simulink model "rtwdemo_sil"  (Simulink 6.0)
settings: Solver=ode3  StartTime=0.0  StopTime=5  FixedStep=.01  RelTol=1e-3
libraries: rtwdemowidgets x1
CloseFcn:
  | rtwprivate ssgencode ModelCloseRequest rtwdemo_sil
settings Model: Creator=The MathWorks Inc.  LastModifiedBy=batserve  ExtModeAutoUpdateStatusClock=off
settings DataIOCC: SaveOutput=off  SaveTime=off  SignalLoggingName=sigsOut
settings OptimizationCC: InlineParams=on  EnforceIntegerDowncast=off  StateBitsets=on  DataBitsets=on  UseTempVars=on  NoFixptDivByZeroProtection=on  LifeSpan=1
settings DebuggingCC: CheckExecutionContextPreStartOutputMsg=on  CheckExecutionContextRuntimeOutputMsg=on  SolverPrmCheckMsg=none
settings RTWCC: SystemTargetFile=ert.tlc  TemplateMakefile=ert_default_tmf  GenerateReport=on  RTWVerbose=off  ProcessScript=ert_make_rtw_hook  IncludeHyperlinkInReport=on  LaunchReport=on
settings CodeAppCC: ForceParamTrailComments=on  IgnoreCustomStorageClasses=off  SimulinkDataObjDesc=on  CustomSymbolStr=$N$M  InsertBlockDesc=on
settings ERTTargetCC: TargetFcnLib=ansi_tfl_tmw.mat  GenFloatMathFcnCalls=ANSI_C  GenerateSampleERTMain=on  IncludeMdlTerminateFcn=off  SupportComplex=off  SupportContinuousTime=on  GenerateErtSFunction=on  InlinedParameterPlacement=NonHierarchical  RootIOFormat=Individual Arguments  ERTCustomFileTemplate=example_file_process.tlc  InitialValueSource=Model

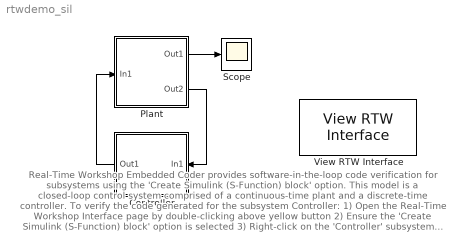
== system rtwdemo_sil ==
  note: Real-Time Workshop Embedded Coder provides software-in-the-loop code verification for subsystems
      | using the 'Create Simulink (S-Function) block' option.  This model is a closed-loop control
      | system comprised of a continuous-time plant and a discrete-time controller.
      |
      | To verify the code generated for the subsystem Controller:
      |
      | 1) Open the Real-Time Workshop Interface page by double-clicking above yellow button
      | 2) Ensure the 'Create Simulink (S-Function) block' option is selected
      | 3) Right-click on the 'Controller' subsystem and select Real-Time Workshop->Build Subsystem...
      | 4) Press the 'Build' button once the parameter dialog appears
      |
      | An S-Function block is created in an untitled library.  This S-Function is a wrapper for the
      | generated subsystem code, and can be used to verify the code provides the same result as the
      | original subsystem.  Replace the original system with the S-Function block and re-run the
      | simulation to verify the output is correct.
  Controller : Subsystem  Orientation=left  TreatAsAtomicUnit=on  PropExecContextAcrossSSBoundary=on
      settings: RTWFcnNameOpts=Use subsystem name  RTWFileNameOpts=Use function name
  Plant : Subsystem  PropExecContextAcrossSSBoundary=on
  Scope : Scope
      settings: TimeRange=5  YMin=0  YMax=10
  View RTW Interface : rtwdemowidgets/View RTW Interface
  wires:
  Controller/1(Out1) -> Plant/1(In1)
  Plant/1(Out1) -> Scope/1
  Plant/2(Out2) -> Controller/1(In1)

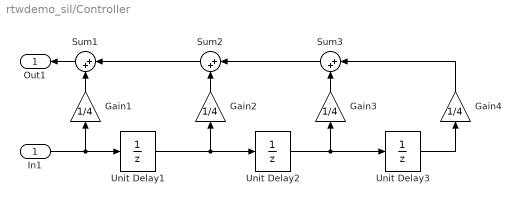
== system rtwdemo_sil/Controller ==
  In1 : Inport  Port=1  SampleTime=.01  LatchInput=off
  Gain{1..4} (4 alike) : Gain  Orientation=up  Gain=1/4  SaturateOnIntegerOverflow=on
  Sum1 : Sum  Orientation=left  Inputs=|++  SaturateOnIntegerOverflow=on  InputSameDT=on
  Sum2 : Sum  Orientation=left  Inputs=|++  SaturateOnIntegerOverflow=on  InputSameDT=on
  Sum3 : Sum  Orientation=left  Inputs=|++  SaturateOnIntegerOverflow=on  InputSameDT=on
  Unit Delay1 : UnitDelay  SampleTime=-1
  Unit Delay2 : UnitDelay  SampleTime=-1
  Unit Delay3 : UnitDelay  SampleTime=-1
  Out1 : Outport  Orientation=left
  wires:
  In1/1 -> Unit Delay1/1, Gain1/1
  Gain2/1 -> Sum2/2
  Gain3/1 -> Sum3/2
  Gain4/1 -> Sum3/1
  Unit Delay3/1 -> Gain4/1
  Unit Delay2/1 -> Gain3/1, Unit Delay3/1
  Unit Delay1/1 -> Gain2/1, Unit Delay2/1
  Sum2/1 -> Sum1/1
  Sum3/1 -> Sum2/1
  Sum1/1 -> Out1/1
  Gain1/1 -> Sum1/2

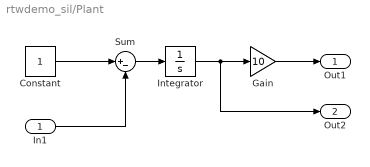
== system rtwdemo_sil/Plant ==
  In1 : Inport  Port=1  LatchInput=off
  Constant : Constant
  Gain : Gain  Gain=10  SaturateOnIntegerOverflow=on
  Integrator : Integrator
  Sum : Sum  Inputs=|+-  SaturateOnIntegerOverflow=on  InputSameDT=on
  Out1 : Outport
  Out2 : Outport  Port=2
  wires:
  Integrator/1 -> Gain/1, Out2/1
  Sum/1 -> Integrator/1
  Constant/1 -> Sum/1
  Gain/1 -> Out1/1
  In1/1 -> Sum/2
